simulink model "M1DCS_2_rust"  (R2020b)
settings: Solver=FixedStepDiscrete  StartTime=0.0  StopTime=5  FixedStep=deltaT  RelTol=1e-3
InitFcn:
  | %
  | % Initialization callback function
  | %
  | 
  | try
  |    fprintf('\n New GMT IMS version!\n');
  | 
  |    % Get Simulink model directory
  |    [filepath,name,ext] = fileparts(which(bdroot));
  | 
  |    if ~strcmp(filepath,pwd)
  |       fprintf('\n Changing current directory to \n %s \n',filepath);
  |       cd(filepath);
  |    end
  | 
  |    %
  |    if(~exist('IMLoads','var'))
  |        warning('Simulation model assumes wind load is loaded...');
  |    end
  | catch
  |    warning('Running the InitFcn from puSimulate script');
  | end
values from neighbouring files (symbols this model uses):
  CS_LC2CG = m1sys{7}.LC2CG    [load_M1DCS_data.m]
  OA_LC2CG = OA_LC2CG + (1/6) * m1sys{i_}.LC2CG    [load_M1DCS_data.m]
  S1_M1RBM2HP = m1sys{1}.M1RBM2HP    [load_M1DCS_data.m]
  S2_M1RBM2HP = m1sys{2}.M1RBM2HP    [load_M1DCS_data.m]
  S3_M1RBM2HP = m1sys{3}.M1RBM2HP    [load_M1DCS_data.m]
  S4_M1RBM2HP = m1sys{4}.M1RBM2HP    [load_M1DCS_data.m]
  S5_M1RBM2HP = m1sys{5}.M1RBM2HP    [load_M1DCS_data.m]
  S6_M1RBM2HP = m1sys{6}.M1RBM2HP    [load_M1DCS_data.m]
  S7_M1RBM2HP = m1sys{7}.M1RBM2HP    [load_M1DCS_data.m]
  SA_dynDen = m1sys{1}.SAdyn.den{1}    [load_M1DCS_data.m]
  SA_dynNum = m1sys{1}.SAdyn.num{1}    [load_M1DCS_data.m]
undefined symbols (not defined in the file or in its folder): dt_SS_struct, m1_HPk, m1sys
libraries: ims_block_library x4
settings Model: SimulationMode=accelerator  Creator=RRomano  LastModifiedBy=rromano
settings DataIOCC: SaveOutput=off  SignalLogging=off  DSMLogging=off  SaveTime=off  ReturnWorkspaceOutputs=off
settings OptimizationCC: DefaultParameterBehavior=Inlined  StrengthReduction=on  PassReuseOutputArgsAs=Individual arguments  EfficientMapNaN2IntZero=off  SimCompilerOptimization=on  AccelVerboseBuild=on  OptimizeBlockOrder=speed  OptimizationPriority=Speed  OptimizationCustomize=off  MultiThreadedLoops=on  EfficientTunableParamExpr=on
settings DebuggingCC: InheritedTsInSrcMsg=none  MultiTaskRateTransMsg=warning  ParameterTunabilityLossMsg=error  SFUnexpectedBacktrackingDiag=warning  SFNoUnconditionalDefaultTransitionDiag=warning  SFExecutionAtInitializationDiag=none  ArithmeticOperatorsInVariantConditions=warning
settings HardwareCC: ProdBitPerLong=64  ProdHWDeviceType=Intel->x86-64 (Linux 64)  TargetBitPerLong=64  TargetBitPerPointer=64  TargetBitPerSizeT=64  TargetBitPerPtrDiffT=64  TargetLongLongMode=on  TargetIntDivRoundTo=Zero  TargetEndianess=LittleEndian  TargetWordSize=64  TargetHWDeviceType=MATLAB Host  ProdEqTarget=off
settings SFSimCC: SimUseLocalCustomCode=off  MATLABDynamicMemAlloc=off  CustomCodeUndefinedFunction=UseInterfaceOnly
settings RTWCC: Description=Embedded Coder  SystemTargetFile=ert.tlc  GenCodeOnly=on  TemplateMakefile=ert_default_tmf  GenerateReport=on  BuildConfiguration=Faster Runs  IncludeHyperlinkInReport=on  GenerateTraceInfo=on  GenerateTraceReport=on  GenerateTraceReportSl=on  GenerateTraceReportSf=on  GenerateTraceReportEml=on
settings CodeAppCC: ForceParamTrailComments=on  IgnoreCustomStorageClasses=off  MaxIdLength=128  OperatorAnnotations=on  SimulinkDataObjDesc=on  SFDataObjDesc=on  InsertBlockDesc=on  MATLABSourceComments=on
settings ERTTargetCC: GenerateSampleERTMain=on  InlinedParameterPlacement=NonHierarchical  ERTCustomFileTemplate=example_file_process.tlc
settings ConfigComp: CovMetricSettings=dw  CovSaveCumulativeToWorkspaceVar=on  CovSaveSingleToWorkspaceVar=on  CovExternalEMLEnable=off

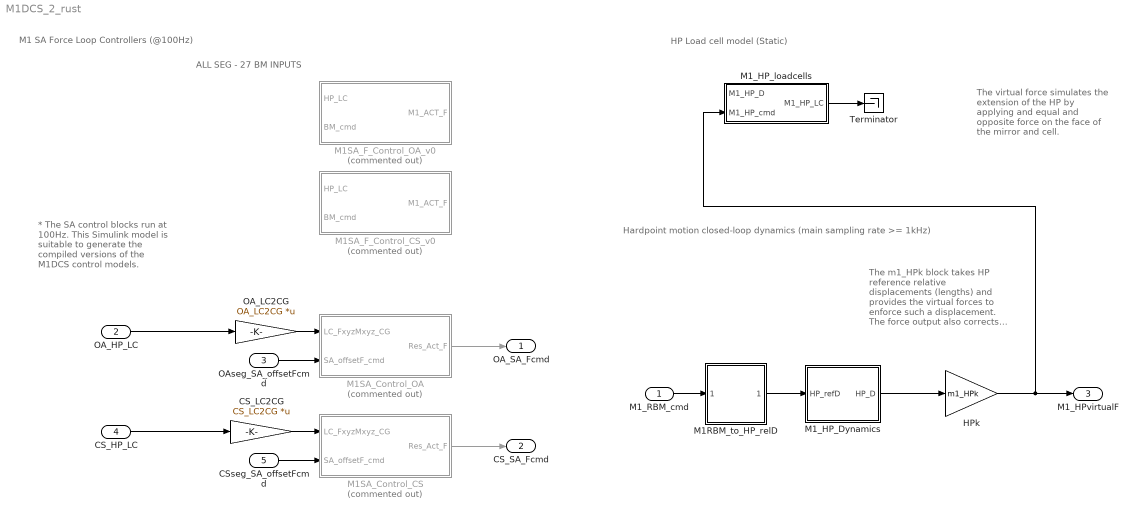
== system M1DCS_2_rust ==
  note: HP Load cell model (Static)
  note: Hardpoint motion closed-loop dynamics (main sampling rate >= 1kHz)
  note: ALL SEG - 27 BM INPUTS
  note: * The SA control blocks run at 100Hz. This Simulink model is suitable to generate the compiled versions of the M1DCS control models.
  note: M1 SA Force Loop Controllers (@100Hz)
  note: The m1_HPk block takes HP reference relative displacements (lengths) and provides the virtual forces to enforce such a displacement. The force output also corrects (offsets) the HP load cell measurement by the commanded change in position.
  note: The virtual force simulates the extension of the HP by applying and equal and opposite force on the face of the mirror and cell.
  M1_RBM_cmd : Inport  PortDimensions=42
  OA_HP_LC : Inport  Port=2  PortDimensions=size(OA_LC2CG,2)  SampleTime=m1sys{1}.ofl.SSdtC{1}.Ts
  OAseg_SA_offsetFcmd : Inport  Port=3  SampleTime=m1sys{1}.ofl.SSdtC{1}.Ts
  CS_HP_LC : Inport  Port=4  PortDimensions=size(CS_LC2CG,2)  SampleTime=m1sys{1}.ofl.SSdtC{1}.Ts
  CSseg_SA_offsetFcmd : Inport  Port=5  SampleTime=m1sys{1}.ofl.SSdtC{1}.Ts
  CS_LC2CG : Gain  Gain=CS_LC2CG  Multiplication=Matrix(K*u)
  HPk : Gain  Gain=m1_HPk
  M1RBM_to_HP_relD : Subsystem
  M1SA_Control_CS : Subsystem  Commented=on
  M1SA_Control_OA : Subsystem  Commented=on
  M1SA_F_Control_CS_v0 : Subsystem  Commented=on
  M1SA_F_Control_OA_v0 : Subsystem  Commented=on
  M1_HP_Dynamics : Subsystem
  M1_HP_loadcells : Subsystem
  OA_LC2CG : Gain  Gain=OA_LC2CG  Multiplication=Matrix(K*u)
  Terminator : Terminator
  OA_SA_Fcmd : Outport  SampleTime=m1sys{1}.ofl.SSdtC{1}.Ts  VectorParamsAs1DForOutWhenUnconnected=off
  CS_SA_Fcmd : Outport  Port=2  SampleTime=m1sys{7}.ofl.SSdtC{1}.Ts  VectorParamsAs1DForOutWhenUnconnected=off
  M1_HPvirtualF : Outport  Port=3  VectorParamsAs1DForOutWhenUnconnected=off
  wires:
  M1_RBM_cmd/1 -> M1RBM_to_HP_relD/1(M1RBM)
  M1SA_Control_CS/1(Res_Act_F) -> CS_SA_Fcmd/1
  CSseg_SA_offsetFcmd/1 -> M1SA_Control_CS/2(SA_offsetF_cmd)
  CS_HP_LC/1 -> CS_LC2CG/1
  M1SA_Control_OA/1(Res_Act_F) -> OA_SA_Fcmd/1
  OA_HP_LC/1 -> OA_LC2CG/1
  OAseg_SA_offsetFcmd/1 -> M1SA_Control_OA/2(SA_offsetF_cmd)
  OA_LC2CG/1 -> M1SA_Control_OA/1(LC_FxyzMxyz_CG)
  CS_LC2CG/1 -> M1SA_Control_CS/1(LC_FxyzMxyz_CG)
  HPk/1 -> M1_HP_loadcells/2(M1_HP_cmd), M1_HPvirtualF/1
  M1RBM_to_HP_relD/1(HP_relD) -> M1_HP_Dynamics/1(HP_refD)
  M1_HP_Dynamics/1(HP_D) -> HPk/1
  M1_HP_loadcells/1(M1_HP_LC) -> Terminator/1

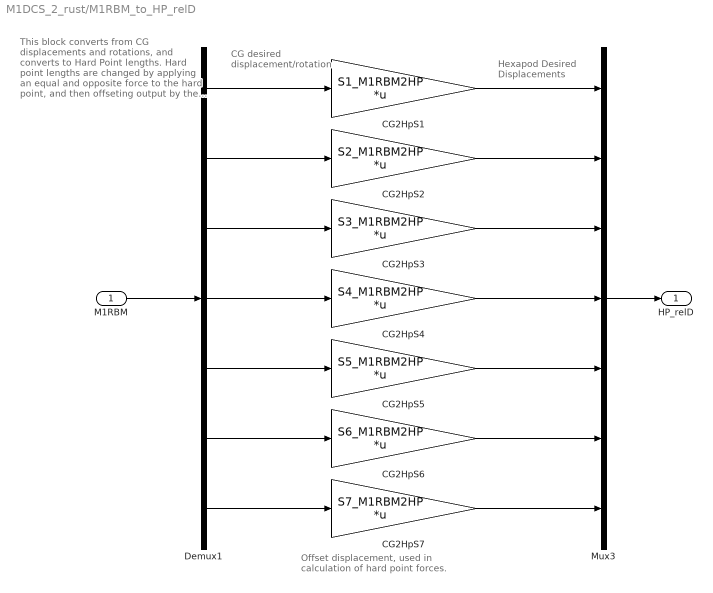
== system M1DCS_2_rust/M1RBM_to_HP_relD ==
  note: CG desired
      | displacement/rotation
  note: This block converts from CG displacements and rotations,
      | and converts to Hard Point lengths.  Hard point lengths are
      | changed by applying an equal and opposite force to the hard
      | point, and then offseting output by the commanded change
      | in position.
  note: Hexapod Desired
      | Displacements
  note: Offset displacement, used in calculation of hard point forces.
  M1RBM : Inport
  CG2HpS1 : Gain  Gain=S1_M1RBM2HP  Multiplication=Matrix(K*u)
  CG2HpS2 : Gain  Gain=S2_M1RBM2HP  Multiplication=Matrix(K*u)
  CG2HpS3 : Gain  Gain=S3_M1RBM2HP  Multiplication=Matrix(K*u)
  CG2HpS4 : Gain  Gain=S4_M1RBM2HP  Multiplication=Matrix(K*u)
  CG2HpS5 : Gain  Gain=S5_M1RBM2HP  Multiplication=Matrix(K*u)
  CG2HpS6 : Gain  Gain=S6_M1RBM2HP  Multiplication=Matrix(K*u)
  CG2HpS7 : Gain  Gain=S7_M1RBM2HP  Multiplication=Matrix(K*u)
  Demux1 : Demux  Outputs=6*ones(7,1)
  Mux3 : Mux  Inputs=6*ones(7,1)
  HP_relD : Outport  VectorParamsAs1DForOutWhenUnconnected=off
  wires:
  Mux3/1 -> HP_relD/1
  Demux1/2 -> CG2HpS2/1
  Demux1/3 -> CG2HpS3/1
  Demux1/4 -> CG2HpS4/1
  Demux1/5 -> CG2HpS5/1
  Demux1/6 -> CG2HpS6/1
  Demux1/1 -> CG2HpS1/1
  Demux1/7 -> CG2HpS7/1
  CG2HpS1/1 -> Mux3/1
  M1RBM/1 -> Demux1/1
  CG2HpS2/1 -> Mux3/2
  CG2HpS3/1 -> Mux3/3
  CG2HpS4/1 -> Mux3/4
  CG2HpS5/1 -> Mux3/5
  CG2HpS6/1 -> Mux3/6
  CG2HpS7/1 -> Mux3/7

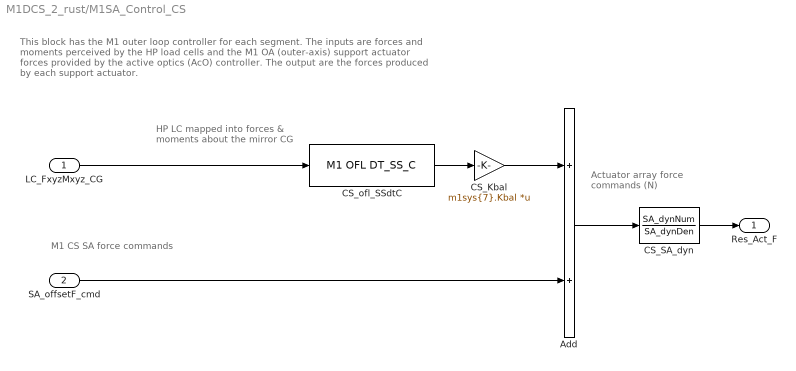
== system M1DCS_2_rust/M1SA_Control_CS ==
  note: This block has the M1 outer loop controller for each segment. The inputs are forces and moments perceived by the HP load cells and the M1 OA (outer-axis) support actuator forces provided by the active optics (AcO) controller. The output are the forces produced by each support actuator.
  note: Actuator array
      | force commands (N)
  note: M1 CS SA
      | force commands
  note: HP LC mapped into forces & moments about the mirror CG
  LC_FxyzMxyz_CG : Inport  PortDimensions=size(m1sys{7}.LC2CG,1)  SampleTime=m1sys{7}.ofl.SSdtC{1}.Ts
  SA_offsetF_cmd : Inport  Port=2  PortDimensions=size(m1sys{7}.Kbal,1)  SampleTime=m1sys{7}.ofl.SSdtC{1}.Ts
  Add : Sum
  CS_Kbal : Gain  Gain=m1sys{7}.Kbal  Multiplication=Matrix(K*u)
  CS_SA_dyn : DiscreteTransferFcn  Numerator=SA_dynNum  Denominator=SA_dynDen  SampleTime=m1sys{7}.ofl.SSdtC{1}.Ts  a0EqualsOne=on
  CS_ofl_SSdtC : ims_block_library/M1 OFL DT_SS_C  dt_SS_struct=CS_ofl_SSdtC
  Res_Act_F : Outport  VectorParamsAs1DForOutWhenUnconnected=off
  wires:
  Add/1 -> CS_SA_dyn/1
  SA_offsetF_cmd/1 -> Add/2
  LC_FxyzMxyz_CG/1 -> CS_ofl_SSdtC/1
  CS_ofl_SSdtC/1 -> CS_Kbal/1
  CS_Kbal/1 -> Add/1
  CS_SA_dyn/1 -> Res_Act_F/1

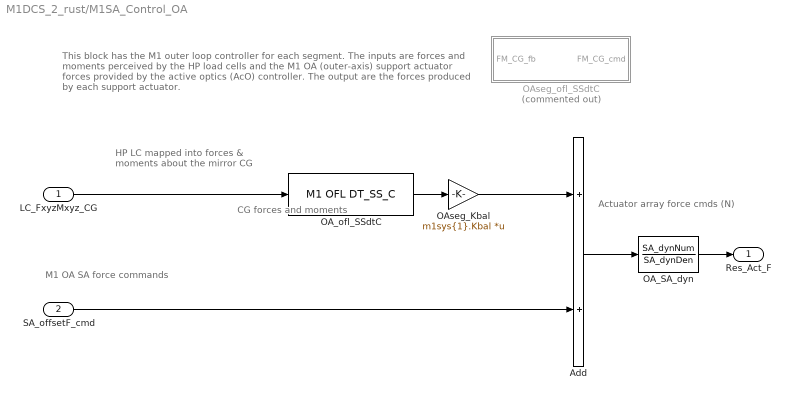
== system M1DCS_2_rust/M1SA_Control_OA ==
  note: M1 OA SA force
      | commands
  note: This block has the M1 outer loop controller for each segment. The inputs are forces and moments perceived by the HP load cells and the M1 OA (outer-axis) support actuator forces provided by the active optics (AcO) controller. The output are the forces produced by each support actuator.
  note: CG forces
      | and moments
  note: Actuator array
      | force cmds (N)
  note: HP LC mapped into forces & moments about the mirror CG
  LC_FxyzMxyz_CG : Inport  PortDimensions=size(m1sys{1}.LC2CG,1)  SampleTime=m1sys{1}.ofl.SSdtC{1}.Ts
  SA_offsetF_cmd : Inport  Port=2  PortDimensions=size(m1sys{1}.Kbal,1)  SampleTime=m1sys{1}.ofl.SSdtC{1}.Ts
  Add : Sum
  OA_SA_dyn : DiscreteTransferFcn  Numerator=SA_dynNum  Denominator=SA_dynDen  SampleTime=m1sys{1}.ofl.SSdtC{1}.Ts  a0EqualsOne=on
  OA_ofl_SSdtC : ims_block_library/M1 OFL DT_SS_C  dt_SS_struct=OA_ofl_SSdtC
  OAseg_Kbal : Gain  Gain=m1sys{1}.Kbal  Multiplication=Matrix(K*u)
  OAseg_ofl_SSdtC : Subsystem  Commented=on  TreatAsAtomicUnit=on
  Res_Act_F : Outport  VectorParamsAs1DForOutWhenUnconnected=off
  wires:
  SA_offsetF_cmd/1 -> Add/2
  OAseg_Kbal/1 -> Add/1
  LC_FxyzMxyz_CG/1 -> OA_ofl_SSdtC/1
  OA_ofl_SSdtC/1 -> OAseg_Kbal/1
  OA_SA_dyn/1 -> Res_Act_F/1
  Add/1 -> OA_SA_dyn/1

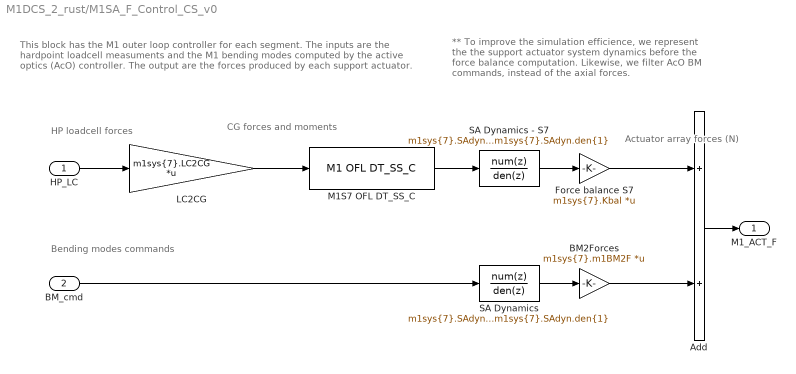
== system M1DCS_2_rust/M1SA_F_Control_CS_v0 ==
  note: This block has the M1 outer loop controller for each segment. The inputs are the hardpoint loadcell measuments and the M1 bending modes computed by the active optics (AcO) controller. The output are the forces produced by each support actuator.
  note: Actuator array
      | forces (N)
  note: HP loadcell
      | forces
  note: ** To improve the simulation efficience, we represent the the support actuator system dynamics before the force balance computation. Likewise, we filter AcO BM commands, instead of the axial forces.
  note: Bending modes
      | commands
  note: CG forces
      | and moments
  HP_LC : Inport  PortDimensions=size(m1sys{7}.LC2CG,1)  SampleTime=m1sys{7}.ofl.SSdtC{1}.Ts
  BM_cmd : Inport  Port=2  PortDimensions=n_bm  SampleTime=m1sys{7}.ofl.SSdtC{1}.Ts
  Add : Sum
  BM2Forces : Gain  Gain=m1sys{7}.m1BM2F  Multiplication=Matrix(K*u)
  Force balance S7 : Gain  Gain=m1sys{7}.Kbal  Multiplication=Matrix(K*u)
  LC2CG : Gain  Gain=m1sys{7}.LC2CG  Multiplication=Matrix(K*u)
  M1S7 OFL DT_SS_C : ims_block_library/M1 OFL DT_SS_C  dt_SS_struct=m1sys{7}.ofl.SSdtC
  SA Dynamics : DiscreteTransferFcn  Numerator=m1sys{7}.SAdyn.num{1}  Denominator=m1sys{7}.SAdyn.den{1}  SampleTime=m1sys{7}.ofl.SSdtC{1}.Ts  a0EqualsOne=on
  SA Dynamics - S7 : DiscreteTransferFcn  Numerator=m1sys{7}.SAdyn.num{1}  Denominator=m1sys{7}.SAdyn.den{1}  SampleTime=m1sys{7}.ofl.SSdtC{1}.Ts  a0EqualsOne=on
  M1_ACT_F : Outport  VectorParamsAs1DForOutWhenUnconnected=off
  wires:
  Force balance S7/1 -> Add/1
  Add/1 -> M1_ACT_F/1
  HP_LC/1 -> LC2CG/1
  SA Dynamics - S7/1 -> Force balance S7/1
  BM2Forces/1 -> Add/2
  M1S7 OFL DT_SS_C/1 -> SA Dynamics - S7/1
  LC2CG/1 -> M1S7 OFL DT_SS_C/1
  BM_cmd/1 -> SA Dynamics/1
  SA Dynamics/1 -> BM2Forces/1

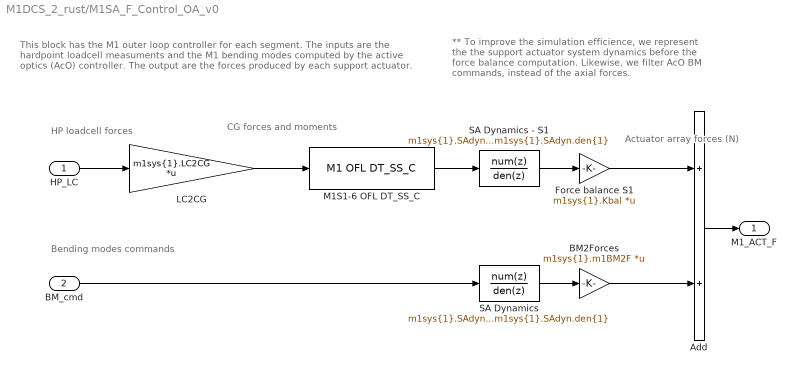
== system M1DCS_2_rust/M1SA_F_Control_OA_v0 ==
  note: ** To improve the simulation efficience, we represent the the support actuator system dynamics before the force balance computation. Likewise, we filter AcO BM commands, instead of the axial forces.
  note: Bending modes
      | commands
  note: This block has the M1 outer loop controller for each segment. The inputs are the hardpoint loadcell measuments and the M1 bending modes computed by the active optics (AcO) controller. The output are the forces produced by each support actuator.
  note: CG forces
      | and moments
  note: Actuator array
      | forces (N)
  note: HP loadcell
      | forces
  HP_LC : Inport  PortDimensions=size(m1sys{1}.LC2CG,1)  SampleTime=m1sys{1}.ofl.SSdtC{1}.Ts
  BM_cmd : Inport  Port=2  PortDimensions=n_bm  SampleTime=m1sys{1}.ofl.SSdtC{1}.Ts
  Add : Sum
  BM2Forces : Gain  Gain=m1sys{1}.m1BM2F  Multiplication=Matrix(K*u)
  Force balance S1 : Gain  Gain=m1sys{1}.Kbal  Multiplication=Matrix(K*u)
  LC2CG : Gain  Gain=m1sys{1}.LC2CG  Multiplication=Matrix(K*u)
  M1S1-6 OFL DT_SS_C : ims_block_library/M1 OFL DT_SS_C  dt_SS_struct=m1sys{1}.ofl.SSdtC
  SA Dynamics : DiscreteTransferFcn  Numerator=m1sys{1}.SAdyn.num{1}  Denominator=m1sys{1}.SAdyn.den{1}  SampleTime=m1sys{1}.ofl.SSdtC{1}.Ts  a0EqualsOne=on
  SA Dynamics - S1 : DiscreteTransferFcn  Numerator=m1sys{1}.SAdyn.num{1}  Denominator=m1sys{1}.SAdyn.den{1}  SampleTime=m1sys{1}.ofl.SSdtC{1}.Ts  a0EqualsOne=on
  M1_ACT_F : Outport  VectorParamsAs1DForOutWhenUnconnected=off
  wires:
  Force balance S1/1 -> Add/1
  M1S1-6 OFL DT_SS_C/1 -> SA Dynamics - S1/1
  HP_LC/1 -> LC2CG/1
  SA Dynamics - S1/1 -> Force balance S1/1
  BM_cmd/1 -> SA Dynamics/1
  LC2CG/1 -> M1S1-6 OFL DT_SS_C/1
  Add/1 -> M1_ACT_F/1
  SA Dynamics/1 -> BM2Forces/1
  BM2Forces/1 -> Add/2

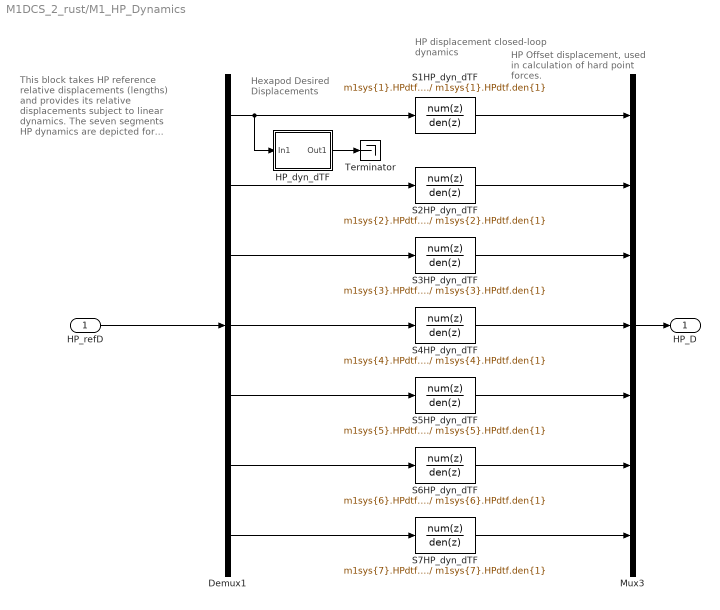
== system M1DCS_2_rust/M1_HP_Dynamics ==
  note: This block takes HP reference relative displacements (lengths) and provides its relative displacements subject to linear dynamics. The seven segments HP dynamics are depicted for illustration. One is supposed to build the single segmen dynamcs ( magenta block HP_dyn_dTF ). Then, the code is cloned for the multiple segments.
  note: Hexapod Desired
      | Displacements
  note: HP Offset displacement, used in calculation of hard point forces.
  note: HP displacement closed-loop dynamics
  HP_refD : Inport
  Demux1 : Demux  Outputs=6*ones(7,1)
  HP_dyn_dTF : Subsystem
  Mux3 : Mux  Inputs=6*ones(7,1)
  S1HP_dyn_dTF : DiscreteTransferFcn  Numerator=m1sys{1}.HPdtf.num{1}  Denominator=m1sys{1}.HPdtf.den{1}  SampleTime=m1sys{1}.HPdtf.Ts  a0EqualsOne=on
  S2HP_dyn_dTF : DiscreteTransferFcn  Numerator=m1sys{2}.HPdtf.num{1}  Denominator=m1sys{2}.HPdtf.den{1}  SampleTime=m1sys{2}.HPdtf.Ts  a0EqualsOne=on
  S3HP_dyn_dTF : DiscreteTransferFcn  Numerator=m1sys{3}.HPdtf.num{1}  Denominator=m1sys{3}.HPdtf.den{1}  SampleTime=m1sys{3}.HPdtf.Ts  a0EqualsOne=on
  S4HP_dyn_dTF : DiscreteTransferFcn  Numerator=m1sys{4}.HPdtf.num{1}  Denominator=m1sys{4}.HPdtf.den{1}  SampleTime=m1sys{4}.HPdtf.Ts  a0EqualsOne=on
  S5HP_dyn_dTF : DiscreteTransferFcn  Numerator=m1sys{5}.HPdtf.num{1}  Denominator=m1sys{5}.HPdtf.den{1}  SampleTime=m1sys{5}.HPdtf.Ts  a0EqualsOne=on
  S6HP_dyn_dTF : DiscreteTransferFcn  Numerator=m1sys{6}.HPdtf.num{1}  Denominator=m1sys{6}.HPdtf.den{1}  SampleTime=m1sys{6}.HPdtf.Ts  a0EqualsOne=on
  S7HP_dyn_dTF : DiscreteTransferFcn  Numerator=m1sys{7}.HPdtf.num{1}  Denominator=m1sys{7}.HPdtf.den{1}  SampleTime=m1sys{7}.HPdtf.Ts  a0EqualsOne=on
  Terminator : Terminator
  HP_D : Outport  VectorParamsAs1DForOutWhenUnconnected=off
  wires:
  Mux3/1 -> HP_D/1
  Demux1/1 -> HP_dyn_dTF/1(In1), S1HP_dyn_dTF/1
  HP_refD/1 -> Demux1/1
  Demux1/2 -> S2HP_dyn_dTF/1
  Demux1/3 -> S3HP_dyn_dTF/1
  Demux1/4 -> S4HP_dyn_dTF/1
  Demux1/5 -> S5HP_dyn_dTF/1
  Demux1/6 -> S6HP_dyn_dTF/1
  Demux1/7 -> S7HP_dyn_dTF/1
  S1HP_dyn_dTF/1 -> Mux3/1
  S2HP_dyn_dTF/1 -> Mux3/2
  S3HP_dyn_dTF/1 -> Mux3/3
  S4HP_dyn_dTF/1 -> Mux3/4
  S5HP_dyn_dTF/1 -> Mux3/5
  S6HP_dyn_dTF/1 -> Mux3/6
  S7HP_dyn_dTF/1 -> Mux3/7
  HP_dyn_dTF/1(Out1) -> Terminator/1

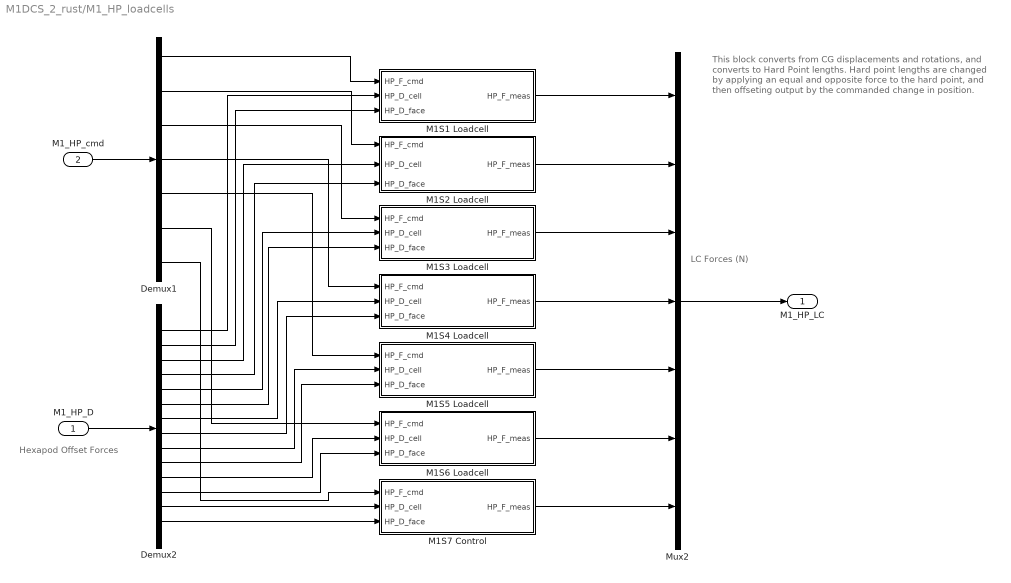
== system M1DCS_2_rust/M1_HP_loadcells ==
  note: This block converts from CG displacements and rotations,
      | and converts to Hard Point lengths.  Hard point lengths are
      | changed by applying an equal and opposite force to the hard
      | point, and then offseting output by the commanded change
      | in position.
  note: Hexapod Offset Forces
  note: LC Forces (N)
  M1_HP_D : Inport
  M1_HP_cmd : Inport  Port=2
  Demux1 : Demux  Outputs=6*ones(7,1)
  Demux2 : Demux  Outputs=6*ones(14,1);%6*ones(7,1)
  M1S1 Loadcell : Subsystem
  M1S2 Loadcell : Subsystem
  M1S3 Loadcell : Subsystem
  M1S4 Loadcell : Subsystem
  M1S5 Loadcell : Subsystem
  M1S6 Loadcell : Subsystem
  M1S7 Control : Subsystem
  Mux2 : Mux  Inputs=7
  M1_HP_LC : Outport  VectorParamsAs1DForOutWhenUnconnected=off
  wires:
  Demux2/9 -> M1S5 Loadcell/2(HP_D_cell)
  Demux2/3 -> M1S2 Loadcell/2(HP_D_cell)
  Demux2/5 -> M1S3 Loadcell/2(HP_D_cell)
  Demux2/13 -> M1S7 Control/2(HP_D_cell)
  Demux2/11 -> M1S6 Loadcell/2(HP_D_cell)
  Demux2/4 -> M1S2 Loadcell/3(HP_D_face)
  Demux2/6 -> M1S3 Loadcell/3(HP_D_face)
  Demux2/10 -> M1S5 Loadcell/3(HP_D_face)
  Demux2/12 -> M1S6 Loadcell/3(HP_D_face)
  Demux2/14 -> M1S7 Control/3(HP_D_face)
  M1_HP_D/1 -> Demux2/1
  M1S1 Loadcell/1(HP_F_meas) -> Mux2/1
  M1S2 Loadcell/1(HP_F_meas) -> Mux2/2
  M1S3 Loadcell/1(HP_F_meas) -> Mux2/3
  M1S5 Loadcell/1(HP_F_meas) -> Mux2/5
  M1S6 Loadcell/1(HP_F_meas) -> Mux2/6
  M1S7 Control/1(HP_F_meas) -> Mux2/7
  Demux2/2 -> M1S1 Loadcell/3(HP_D_face)
  Demux2/1 -> M1S1 Loadcell/2(HP_D_cell)
  M1S4 Loadcell/1(HP_F_meas) -> Mux2/4
  Demux2/7 -> M1S4 Loadcell/2(HP_D_cell)
  Demux2/8 -> M1S4 Loadcell/3(HP_D_face)
  M1_HP_cmd/1 -> Demux1/1
  Demux1/1 -> M1S1 Loadcell/1(HP_F_cmd)
  Demux1/2 -> M1S2 Loadcell/1(HP_F_cmd)
  Demux1/3 -> M1S3 Loadcell/1(HP_F_cmd)
  Demux1/4 -> M1S4 Loadcell/1(HP_F_cmd)
  Demux1/5 -> M1S5 Loadcell/1(HP_F_cmd)
  Demux1/6 -> M1S6 Loadcell/1(HP_F_cmd)
  Demux1/7 -> M1S7 Control/1(HP_F_cmd)
  Mux2/1 -> M1_HP_LC/1

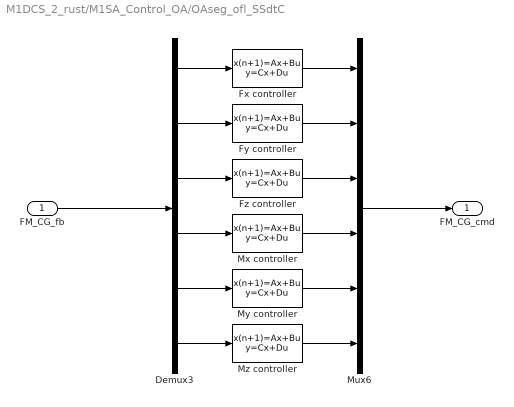
== system M1DCS_2_rust/M1SA_Control_OA/OAseg_ofl_SSdtC ==
  FM_CG_fb : Inport
  Demux3 : Demux  Outputs=6
  Fx controller : DiscreteStateSpace  A=dt_SS_struct{1}.A  B=dt_SS_struct{1}.B  C=dt_SS_struct{1}.C  D=dt_SS_struct{1}.D  SampleTime=dt_SS_struct{1}.Ts
  Fy controller : DiscreteStateSpace  A=dt_SS_struct{2}.A  B=dt_SS_struct{2}.B  C=dt_SS_struct{2}.C  D=dt_SS_struct{2}.D  SampleTime=dt_SS_struct{2}.Ts
  Fz controller : DiscreteStateSpace  A=dt_SS_struct{3}.A  B=dt_SS_struct{3}.B  C=dt_SS_struct{3}.C  D=dt_SS_struct{3}.D  SampleTime=dt_SS_struct{3}.Ts
  Mux6 : Mux  Inputs=6
  Mx controller : DiscreteStateSpace  A=dt_SS_struct{4}.A  B=dt_SS_struct{4}.B  C=dt_SS_struct{4}.C  D=dt_SS_struct{4}.D  SampleTime=dt_SS_struct{4}.Ts
  My controller : DiscreteStateSpace  A=dt_SS_struct{5}.A  B=dt_SS_struct{5}.B  C=dt_SS_struct{5}.C  D=dt_SS_struct{5}.D  SampleTime=dt_SS_struct{5}.Ts
  Mz controller : DiscreteStateSpace  A=dt_SS_struct{6}.A  B=dt_SS_struct{6}.B  C=dt_SS_struct{6}.C  D=dt_SS_struct{6}.D  SampleTime=dt_SS_struct{6}.Ts
  FM_CG_cmd : Outport  VectorParamsAs1DForOutWhenUnconnected=off
  wires:
  Fz controller/1 -> Mux6/3
  Demux3/6 -> Mz controller/1
  Mux6/1 -> FM_CG_cmd/1
  Demux3/2 -> Fy controller/1
  Mz controller/1 -> Mux6/6
  Demux3/4 -> Mx controller/1
  Demux3/3 -> Fz controller/1
  FM_CG_fb/1 -> Demux3/1
  Fy controller/1 -> Mux6/2
  Fx controller/1 -> Mux6/1
  Mx controller/1 -> Mux6/4
  Demux3/5 -> My controller/1
  My controller/1 -> Mux6/5
  Demux3/1 -> Fx controller/1

== system M1DCS_2_rust/M1_HP_Dynamics/HP_dyn_dTF ==
  In1 : Inport
  HP_dyn_dTF : DiscreteTransferFcn  Numerator=m1sys{1}.HPdtf.num{1}  Denominator=m1sys{1}.HPdtf.den{1}  SampleTime=m1sys{1}.HPdtf.Ts  a0EqualsOne=on
  Out1 : Outport
  wires:
  HP_dyn_dTF/1 -> Out1/1
  In1/1 -> HP_dyn_dTF/1

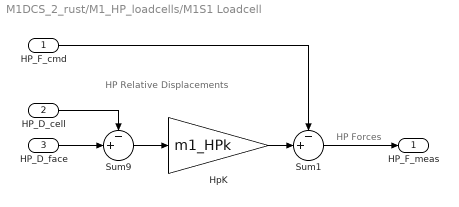
== system M1DCS_2_rust/M1_HP_loadcells/M1S1 Loadcell ==
  note: HP Forces
  note: HP Relative
      | Displacements
  HP_F_cmd : Inport
  HP_D_cell : Inport  Port=2
  HP_D_face : Inport  Port=3
  HpK : Gain  Gain=m1_HPk
  Sum1 : Sum  Inputs=-+|
  Sum9 : Sum  Inputs=-+|
  HP_F_meas : Outport  VectorParamsAs1DForOutWhenUnconnected=off
  wires:
  HP_D_cell/1 -> Sum9/1
  HP_D_face/1 -> Sum9/2
  Sum9/1 -> HpK/1
  HpK/1 -> Sum1/2
  Sum1/1 -> HP_F_meas/1
  HP_F_cmd/1 -> Sum1/1

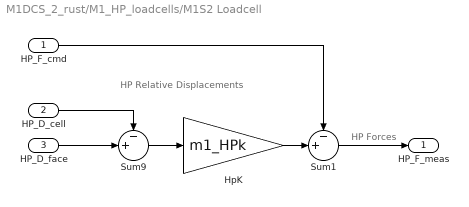
== system M1DCS_2_rust/M1_HP_loadcells/M1S2 Loadcell ==
  note: HP Relative
      | Displacements
  note: HP Forces
  HP_F_cmd : Inport
  HP_D_cell : Inport  Port=2
  HP_D_face : Inport  Port=3
  HpK : Gain  Gain=m1_HPk
  Sum1 : Sum  Inputs=-+|
  Sum9 : Sum  Inputs=-+|
  HP_F_meas : Outport  VectorParamsAs1DForOutWhenUnconnected=off
  wires:
  HP_D_face/1 -> Sum9/2
  HP_D_cell/1 -> Sum9/1
  HP_F_cmd/1 -> Sum1/1
  HpK/1 -> Sum1/2
  Sum1/1 -> HP_F_meas/1
  Sum9/1 -> HpK/1

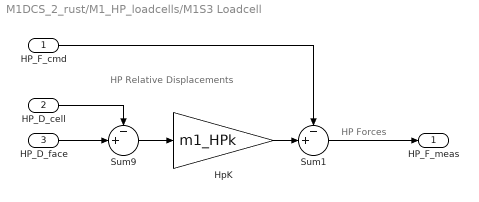
== system M1DCS_2_rust/M1_HP_loadcells/M1S3 Loadcell ==
  note: HP Relative
      | Displacements
  note: HP Forces
  HP_F_cmd : Inport
  HP_D_cell : Inport  Port=2
  HP_D_face : Inport  Port=3
  HpK : Gain  Gain=m1_HPk
  Sum1 : Sum  Inputs=-+|
  Sum9 : Sum  Inputs=-+|
  HP_F_meas : Outport  VectorParamsAs1DForOutWhenUnconnected=off
  wires:
  HP_D_face/1 -> Sum9/2
  HP_D_cell/1 -> Sum9/1
  HP_F_cmd/1 -> Sum1/1
  HpK/1 -> Sum1/2
  Sum1/1 -> HP_F_meas/1
  Sum9/1 -> HpK/1

== system M1DCS_2_rust/M1_HP_loadcells/M1S4 Loadcell ==
  note: HP Relative
      | Displacements
  note: HP Forces
  HP_F_cmd : Inport
  HP_D_cell : Inport  Port=2
  HP_D_face : Inport  Port=3
  HpK : Gain  Gain=m1_HPk
  Sum1 : Sum  Inputs=-+|
  Sum9 : Sum  Inputs=-+|
  HP_F_meas : Outport  VectorParamsAs1DForOutWhenUnconnected=off
  wires:
  HP_D_face/1 -> Sum9/2
  HP_D_cell/1 -> Sum9/1
  HP_F_cmd/1 -> Sum1/1
  HpK/1 -> Sum1/2
  Sum1/1 -> HP_F_meas/1
  Sum9/1 -> HpK/1

== system M1DCS_2_rust/M1_HP_loadcells/M1S5 Loadcell ==
  note: HP Relative
      | Displacements
  note: HP Forces
  HP_F_cmd : Inport
  HP_D_cell : Inport  Port=2
  HP_D_face : Inport  Port=3
  HpK : Gain  Gain=m1_HPk
  Sum1 : Sum  Inputs=-+|
  Sum9 : Sum  Inputs=-+|
  HP_F_meas : Outport  VectorParamsAs1DForOutWhenUnconnected=off
  wires:
  HP_D_face/1 -> Sum9/2
  HP_D_cell/1 -> Sum9/1
  HP_F_cmd/1 -> Sum1/1
  HpK/1 -> Sum1/2
  Sum1/1 -> HP_F_meas/1
  Sum9/1 -> HpK/1

== system M1DCS_2_rust/M1_HP_loadcells/M1S6 Loadcell ==
  note: HP Relative
      | Displacements
  note: HP Forces
  HP_F_cmd : Inport
  HP_D_cell : Inport  Port=2
  HP_D_face : Inport  Port=3
  HpK : Gain  Gain=m1_HPk
  Sum1 : Sum  Inputs=-+|
  Sum9 : Sum  Inputs=-+|
  HP_F_meas : Outport  VectorParamsAs1DForOutWhenUnconnected=off
  wires:
  HP_D_face/1 -> Sum9/2
  HP_D_cell/1 -> Sum9/1
  HP_F_cmd/1 -> Sum1/1
  HpK/1 -> Sum1/2
  Sum1/1 -> HP_F_meas/1
  Sum9/1 -> HpK/1

== system M1DCS_2_rust/M1_HP_loadcells/M1S7 Control ==
  note: HP Relative
      | Displacements
  note: HP Forces
  HP_F_cmd : Inport
  HP_D_cell : Inport  Port=2
  HP_D_face : Inport  Port=3
  HpK : Gain  Gain=m1_HPk
  Sum1 : Sum  Inputs=-+|
  Sum9 : Sum  Inputs=-+|
  HP_F_meas : Outport  VectorParamsAs1DForOutWhenUnconnected=off
  wires:
  HP_D_face/1 -> Sum9/2
  HP_D_cell/1 -> Sum9/1
  HP_F_cmd/1 -> Sum1/1
  HpK/1 -> Sum1/2
  Sum1/1 -> HP_F_meas/1
  Sum9/1 -> HpK/1
